simulink model "MyModule5_WaterTank"  (R2021b)
settings: Solver=ode4  StartTime=0.0  StopTime=5000  RelTol=1e-3
undefined symbols (not defined in the file): A1, A2, A3, c0, c1, c2, k, simSwitch, x0
settings Model: Creator=tanzc  LastModifiedBy=tanzc
settings SolverCC: AlgebraicLoopSolver=TrustRegion
settings DataIOCC: ExternalInput=[0 5 5]  InitialState=[]  LoadExternalInput=on  LoadInitialState=on  SaveFormat=Structure  ReturnWorkspaceOutputs=off  StateSaveName=x  TimeSaveName=t  OutputSaveName=y
settings OptimizationCC: DefaultParameterBehavior=Inlined  BufferReuse=off
settings DebuggingCC: InitInArrayFormatMsg=none  SFMachineParentedDataDiag=warning

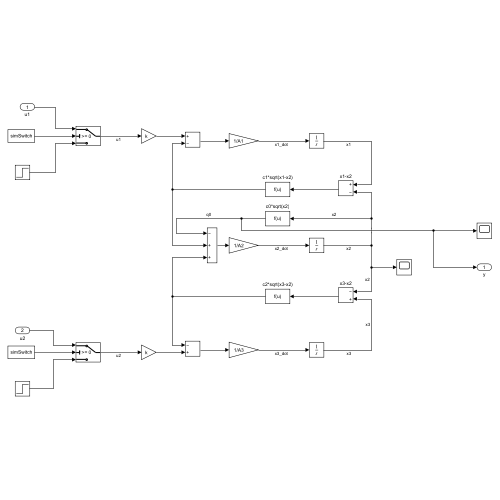
[thumbnail: Simulink's stored preview of the top-level diagram]
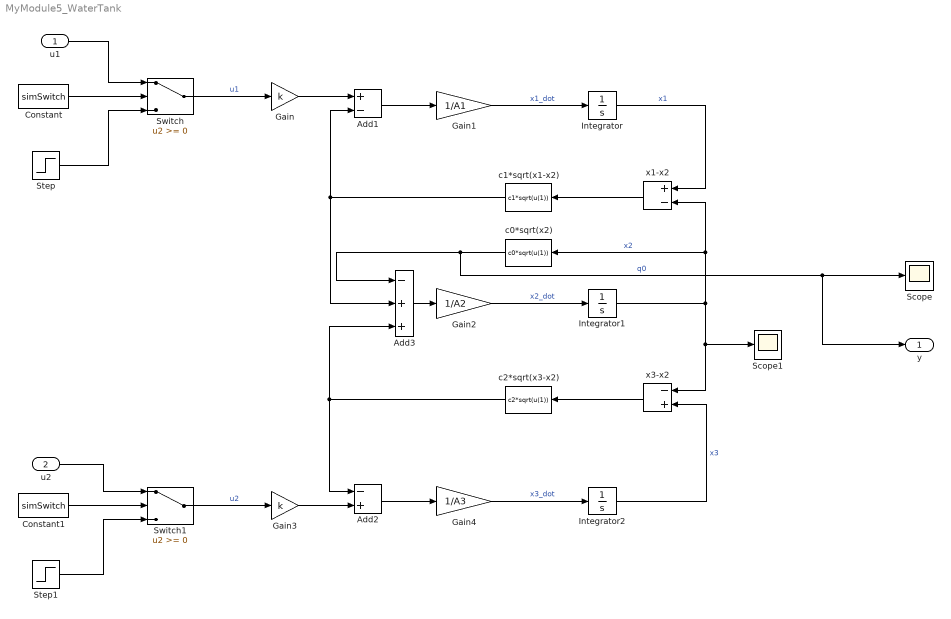
== system MyModule5_WaterTank ==
  u1 : Inport
  u2 : Inport  Port=2
  Add1 : Sum  Inputs=+-
  Add2 : Sum  Inputs=-+
  Add3 : Sum  Inputs=-++
  Constant : Constant  Value=simSwitch
  Constant1 : Constant  Value=simSwitch
  Gain : Gain  Gain=k
  Gain1 : Gain  Gain=1/A1
  Gain2 : Gain  Gain=1/A2
  Gain3 : Gain  Gain=k
  Gain4 : Gain  Gain=1/A3
  Integrator : Integrator  Priority=1  InitialCondition=x0(1)
  Integrator1 : Integrator  Priority=2  InitialCondition=x0(2)
  Integrator2 : Integrator  Priority=3  InitialCondition=x0(3)
  Scope : Scope
  Scope1 : Scope
  Step : Step  Time=0  Before=u  After=u  SampleTime=0.1
  Step1 : Step  Time=0  Before=u  After=u  SampleTime=0.1
  Switch : Switch
  Switch1 : Switch
  c0*sqrt(x2) : Fcn  Expr=c0*sqrt(u(1))
  c1*sqrt(x1-x2) : Fcn  Expr=c1*sqrt(u(1))
  c2*sqrt(x3-x2) : Fcn  Expr=c2*sqrt(u(1))
  x1-x2 : Sum  Inputs=+-
  x3-x2 : Sum  Inputs=-+
  y : Outport
  wires:
  u2/1 -> Switch1/1
  x3-x2/1 -> c2*sqrt(x3-x2)/1
  Integrator2/1 -> x3-x2/2  "x3"
  Gain/1 -> Add1/1
  c1*sqrt(x1-x2)/1 -> Add3/2, Add1/2
  c2*sqrt(x3-x2)/1 -> Add2/1, Add3/3
  Integrator/1 -> x1-x2/1  "x1"
  Step/1 -> Switch/3
  Add1/1 -> Gain1/1
  Gain1/1 -> Integrator/1  "x1_dot"
  Switch/1 -> Gain/1  "u1"
  Add3/1 -> Gain2/1
  Gain4/1 -> Integrator2/1  "x3_dot"
  x1-x2/1 -> c1*sqrt(x1-x2)/1
  c0*sqrt(x2)/1 -> y/1, Scope/1, Add3/1  "q0"
  Switch1/1 -> Gain3/1  "u2"
  Constant/1 -> Switch/2
  Gain2/1 -> Integrator1/1  "x2_dot"
  Gain3/1 -> Add2/2
  Add2/1 -> Gain4/1
  Integrator1/1 -> Scope1/1, x3-x2/1, c0*sqrt(x2)/1, x1-x2/2  "x2"
  Step1/1 -> Switch1/3
  Constant1/1 -> Switch1/2
  u1/1 -> Switch/1
